simulink model "model"  (R2014a)
(part 8 of 8)

  _CN_242253500_500000_CN_204258596_500000/RConn3 -- T_204258596_500000_/LConn3 -- 関門連系線_CN_204258596_500000_CN_187988970_500000/RConn3 -- _CN_204258596_500000_CN_317416612_500000/RConn3 -- bus260/LConn1
  T_216956620_500000_/LConn1 -- 小丸川幹線_CN_216956620_500000_CN_216953915_220000/RConn1
  T_216956620_500000_/LConn2 -- 小丸川幹線_CN_216956620_500000_CN_216953915_220000/RConn2
  小丸川幹線_CN_216956620_500000_CN_216953915_220000/RConn3 -- T_216956620_500000_/LConn3 -- bus261/LConn1
  _CN_253566674_500000_CN_156208858_500000/LConn1 -- T_253566674__/LConn1 -- _CN_253566674_500000_CN_104391636_500000/LConn1
  _CN_253566674_500000_CN_156208858_500000/LConn2 -- T_253566674__/LConn2 -- _CN_253566674_500000_CN_104391636_500000/LConn2
  _CN_253566674_500000_CN_156208858_500000/LConn3 -- T_253566674__/LConn3 -- _CN_253566674_500000_CN_104391636_500000/LConn3 -- bus262/LConn1
  T_156208858_500000_南相馬変電所/LConn1 -- _CN_253566674_500000_CN_156208858_500000/RConn1
  T_156208858_500000_南相馬変電所/LConn2 -- _CN_253566674_500000_CN_156208858_500000/RConn2
  _CN_253566674_500000_CN_156208858_500000/RConn3 -- T_156208858_500000_南相馬変電所/LConn3 -- bus263/LConn1
  _CN_253566674_500000_CN_104391636_500000/RConn1 -- T_104391636_500000_新いわき/LConn1 -- 福島東幹線2_CN_106309481_500000_CN_104391636_500000/RConn1 -- _CN_132913106_500000_CN_104391636_500000/RConn1 -- 福島幹線_CN_104391636_500000_CN_168839127_500000/RConn1
  _CN_253566674_500000_CN_104391636_500000/RConn2 -- T_104391636_500000_新いわき/LConn2 -- 福島東幹線2_CN_106309481_500000_CN_104391636_500000/RConn2 -- _CN_132913106_500000_CN_104391636_500000/RConn2 -- 福島幹線_CN_104391636_500000_CN_168839127_500000/RConn2
  _CN_253566674_500000_CN_104391636_500000/RConn3 -- T_104391636_500000_新いわき/LConn3 -- 福島東幹線2_CN_106309481_500000_CN_104391636_500000/RConn3 -- _CN_132913106_500000_CN_104391636_500000/RConn3 -- 福島幹線_CN_104391636_500000_CN_168839127_500000/RConn3 -- bus264/LConn1
  新榛名線_CN_169963227_500000_CN_195615141_500000/LConn1 -- T_169963227_500000_新榛名/LConn1 -- _CN_169963227_500000_CN_169963236_500000/LConn1
  新榛名線_CN_169963227_500000_CN_195615141_500000/LConn2 -- T_169963227_500000_新榛名/LConn2 -- _CN_169963227_500000_CN_169963236_500000/LConn2
  新榛名線_CN_169963227_500000_CN_195615141_500000/LConn3 -- T_169963227_500000_新榛名/LConn3 -- _CN_169963227_500000_CN_169963236_500000/LConn3 -- bus265/LConn1
  新榛名線_CN_169963227_500000_CN_195615141_500000/RConn1 -- T_195615141_500000_/LConn1 -- _CN_195615141_500000_CN_315662839_500000/LConn1
  新榛名線_CN_169963227_500000_CN_195615141_500000/RConn2 -- T_195615141_500000_/LConn2 -- _CN_195615141_500000_CN_315662839_500000/LConn2
  新榛名線_CN_169963227_500000_CN_195615141_500000/RConn3 -- T_195615141_500000_/LConn3 -- _CN_195615141_500000_CN_315662839_500000/LConn3 -- bus266/LConn1
  _CN_169963227_500000_CN_169963236_500000/RConn1 -- T_169963236__/LConn1 -- 新吾妻線_CN_169963236_500000_CN_66098469_500000/RConn1
  _CN_169963227_500000_CN_169963236_500000/RConn2 -- T_169963236__/LConn2 -- 新吾妻線_CN_169963236_500000_CN_66098469_500000/RConn2
  _CN_169963227_500000_CN_169963236_500000/RConn3 -- T_169963236__/LConn3 -- 新吾妻線_CN_169963236_500000_CN_66098469_500000/RConn3 -- bus267/LConn1
  T_242103532_500000_/LConn1 -- _CN_242103532_500000_CN_241822623_500000/LConn1
  T_242103532_500000_/LConn2 -- _CN_242103532_500000_CN_241822623_500000/LConn2
  _CN_242103532_500000_CN_241822623_500000/LConn3 -- T_242103532_500000_/LConn3 -- bus268/LConn1
  _CN_242103532_500000_CN_241822623_500000/RConn1 -- T_241822623_500000;220000;110000_/LConn1 -- _CN_241822623_500000_CN_241822631_500000/LConn1 -- _CN_241828221_500000_CN_241822623_500000/RConn1
  _CN_242103532_500000_CN_241822623_500000/RConn2 -- T_241822623_500000;220000;110000_/LConn2 -- _CN_241822623_500000_CN_241822631_500000/LConn2 -- _CN_241828221_500000_CN_241822623_500000/RConn2
  _CN_242103532_500000_CN_241822623_500000/RConn3 -- T_241822623_500000;220000;110000_/LConn3 -- _CN_241822623_500000_CN_241822631_500000/LConn3 -- bus269/LConn1 -- _CN_241828221_500000_CN_241822623_500000/RConn3
  T_169031922__/LConn1 -- _CN_169031922_500000_CN_169031998_500000/LConn1
  T_169031922__/LConn2 -- _CN_169031922_500000_CN_169031998_500000/LConn2
  _CN_169031922_500000_CN_169031998_500000/LConn3 -- T_169031922__/LConn3 -- bus270/LConn1
  _CN_169031922_500000_CN_169031998_500000/RConn1 -- T_169031998__/LConn1 -- _CN_169031998_500000_CN_109850439_500000/LConn1 -- _CN_169031998_500000_CN_161870227_500000/RConn1
  _CN_169031922_500000_CN_169031998_500000/RConn2 -- T_169031998__/LConn2 -- _CN_169031998_500000_CN_109850439_500000/LConn2 -- _CN_169031998_500000_CN_161870227_500000/RConn2
  _CN_169031922_500000_CN_169031998_500000/RConn3 -- T_169031998__/LConn3 -- _CN_169031998_500000_CN_109850439_500000/LConn3 -- _CN_169031998_500000_CN_161870227_500000/RConn3 -- bus271/LConn1
  T_250540807_500000_東群馬変電所_(Higashi_Gunma_Substation)/LConn1 -- 東群馬幹線_CN_250540807_500000_CN_66098469_500000/RConn1
  T_250540807_500000_東群馬変電所_(Higashi_Gunma_Substation)/LConn2 -- 東群馬幹線_CN_250540807_500000_CN_66098469_500000/RConn2
  東群馬幹線_CN_250540807_500000_CN_66098469_500000/RConn3 -- T_250540807_500000_東群馬変電所_(Higashi_Gunma_Substation)/LConn3 -- bus272/LConn1
  T_151379730_500000_房総変電所_(Bōsō_Hendensho)/LConn1 -- 房総線_CN_151379730_500000_CN_168727982_500000/RConn1
  T_151379730_500000_房総変電所_(Bōsō_Hendensho)/LConn2 -- 房総線_CN_151379730_500000_CN_168727982_500000/RConn2
  房総線_CN_151379730_500000_CN_168727982_500000/RConn3 -- T_151379730_500000_房総変電所_(Bōsō_Hendensho)/LConn3 -- bus273/LConn1
  南信幹線_CN_142662111_500000_CN_209429410_500000/RConn1 -- T_209429410_500000_南信変電所/LConn1 -- 信濃幹線_CN_209726348_500000_CN_209429410_500000/LConn1
  南信幹線_CN_142662111_500000_CN_209429410_500000/RConn2 -- T_209429410_500000_南信変電所/LConn2 -- 信濃幹線_CN_209726348_500000_CN_209429410_500000/LConn2
  南信幹線_CN_142662111_500000_CN_209429410_500000/RConn3 -- T_209429410_500000_南信変電所/LConn3 -- 信濃幹線_CN_209726348_500000_CN_209429410_500000/LConn3 -- bus274/LConn1
  T_106076988_500000_宮城変電所/LConn1 -- _CN_106076988_500000_CN_174636874_500000/LConn1
  T_106076988_500000_宮城変電所/LConn2 -- _CN_106076988_500000_CN_174636874_500000/LConn2
  _CN_106076988_500000_CN_174636874_500000/LConn3 -- T_106076988_500000_宮城変電所/LConn3 -- bus275/LConn1
  T_174636874_275000_岩手変電所/LConn1 -- _CN_106076988_500000_CN_174636874_500000/RConn1
  T_174636874_275000_岩手変電所/LConn2 -- _CN_106076988_500000_CN_174636874_500000/RConn2
  _CN_106076988_500000_CN_174636874_500000/RConn3 -- T_174636874_275000_岩手変電所/LConn3 -- bus276/LConn1
  _CN_169031998_500000_CN_109850439_500000/RConn1 -- T_109850439_500000_/LConn1 -- 阿南紀北直流幹線_CN_109850439_500000_CN_217885658_500000/LConn1
  _CN_169031998_500000_CN_109850439_500000/RConn2 -- T_109850439_500000_/LConn2 -- 阿南紀北直流幹線_CN_109850439_500000_CN_217885658_500000/LConn2
  _CN_169031998_500000_CN_109850439_500000/RConn3 -- T_109850439_500000_/LConn3 -- 阿南紀北直流幹線_CN_109850439_500000_CN_217885658_500000/LConn3 -- bus277/LConn1
  新筑波線_(Shin_Tsukuba_Sen)_CN_133135172_500000_CN_132913106_500000/RConn1 -- T_133135172_500000_新古河変電所/LConn1 -- 新京葉線_CN_133135172_500000_CN_168727982_500000/RConn1 -- 新京葉線_CN_133135172_500000_CN_151706977_500000/LConn1 -- 新古河線_(Shin_Koga_Sen)_CN_133135172_500000_CN_133641619_500000/RConn1 -- 福島幹線_CN_133135172_500000_CN_168839127_500000/RConn1
  新筑波線_(Shin_Tsukuba_Sen)_CN_133135172_500000_CN_132913106_500000/RConn2 -- T_133135172_500000_新古河変電所/LConn2 -- 新京葉線_CN_133135172_500000_CN_168727982_500000/RConn2 -- 新京葉線_CN_133135172_500000_CN_151706977_500000/LConn2 -- 新古河線_(Shin_Koga_Sen)_CN_133135172_500000_CN_133641619_500000/RConn2 -- 福島幹線_CN_133135172_500000_CN_168839127_500000/RConn2
  新筑波線_(Shin_Tsukuba_Sen)_CN_133135172_500000_CN_132913106_500000/RConn3 -- T_133135172_500000_新古河変電所/LConn3 -- 新京葉線_CN_133135172_500000_CN_168727982_500000/RConn3 -- 新京葉線_CN_133135172_500000_CN_151706977_500000/LConn3 -- 新古河線_(Shin_Koga_Sen)_CN_133135172_500000_CN_133641619_500000/RConn3 -- 福島幹線_CN_133135172_500000_CN_168839127_500000/RConn3 -- bus278/LConn1
  T_151706977__新野田変電所_(Shin_Noda_Hendensho)/LConn1 -- 新京葉線_CN_133135172_500000_CN_151706977_500000/RConn1
  T_151706977__新野田変電所_(Shin_Noda_Hendensho)/LConn2 -- 新京葉線_CN_133135172_500000_CN_151706977_500000/RConn2
  新京葉線_CN_133135172_500000_CN_151706977_500000/RConn3 -- T_151706977__新野田変電所_(Shin_Noda_Hendensho)/LConn3 -- bus279/LConn1
  T_217885658_500000;0_由良開閉所/LConn1 -- 阿南紀北直流幹線_CN_109850439_500000_CN_217885658_500000/RConn1
  T_217885658_500000;0_由良開閉所/LConn2 -- 阿南紀北直流幹線_CN_109850439_500000_CN_217885658_500000/RConn2
  阿南紀北直流幹線_CN_109850439_500000_CN_217885658_500000/RConn3 -- T_217885658_500000;0_由良開閉所/LConn3 -- bus280/LConn1
  T_185029969_500000;220000_/LConn1 -- _CN_185029969_500000_CN_216798219_500000/LConn1
  T_185029969_500000;220000_/LConn2 -- _CN_185029969_500000_CN_216798219_500000/LConn2
  _CN_185029969_500000_CN_216798219_500000/LConn3 -- T_185029969_500000;220000_/LConn3 -- bus281/LConn1
  G_216798219_九州電力_松浦火力発電所/RConn1 -- _CN_185029969_500000_CN_216798219_500000/RConn1
  G_216798219_九州電力_松浦火力発電所/RConn2 -- _CN_185029969_500000_CN_216798219_500000/RConn2
  _CN_185029969_500000_CN_216798219_500000/RConn3 -- G_216798219_九州電力_松浦火力発電所/RConn3 -- bus282/LConn1
  _CN_170605907_500000_CN_110682956_500000/RConn1 -- T_170605907_500000_北摂変電所/LConn1 -- _CN_170605907_500000_CN_241822631_500000/LConn1
  _CN_170605907_500000_CN_110682956_500000/RConn2 -- T_170605907_500000_北摂変電所/LConn2 -- _CN_170605907_500000_CN_241822631_500000/LConn2
  _CN_170605907_500000_CN_110682956_500000/RConn3 -- T_170605907_500000_北摂変電所/LConn3 -- _CN_170605907_500000_CN_241822631_500000/LConn3 -- bus283/LConn1
  _CN_170605907_500000_CN_241822631_500000/RConn1 -- T_241822631__/LConn1 -- _CN_241822623_500000_CN_241822631_500000/RConn1 -- _CN_241822621_500000_CN_241822631_500000/RConn1
  _CN_170605907_500000_CN_241822631_500000/RConn2 -- T_241822631__/LConn2 -- _CN_241822623_500000_CN_241822631_500000/RConn2 -- _CN_241822621_500000_CN_241822631_500000/RConn2
  _CN_170605907_500000_CN_241822631_500000/RConn3 -- T_241822631__/LConn3 -- _CN_241822623_500000_CN_241822631_500000/RConn3 -- bus284/LConn1 -- _CN_241822621_500000_CN_241822631_500000/RConn3
  T_209726348_500000_信濃変電所/LConn1 -- 信濃幹線_CN_209726348_500000_CN_209429410_500000/RConn1
  T_209726348_500000_信濃変電所/LConn2 -- 信濃幹線_CN_209726348_500000_CN_209429410_500000/RConn2
  信濃幹線_CN_209726348_500000_CN_209429410_500000/RConn3 -- T_209726348_500000_信濃変電所/LConn3 -- bus285/LConn1
  T_315662839_500000_新信濃変電所/LConn1 -- _CN_195615141_500000_CN_315662839_500000/RConn1
  T_315662839_500000_新信濃変電所/LConn2 -- _CN_195615141_500000_CN_315662839_500000/RConn2
  _CN_195615141_500000_CN_315662839_500000/RConn3 -- T_315662839_500000_新信濃変電所/LConn3 -- bus286/LConn1
  T_259056356__/RConn1 -- L_259056356/LConn1
  T_259056356__/RConn2 -- L_259056356/LConn2
  L_259056356/LConn3 -- T_259056356__/RConn3 -- bus287/LConn1
  T_90806466_220000;66000_/RConn1 -- L_90806466/LConn1
  T_90806466_220000;66000_/RConn2 -- L_90806466/LConn2
  L_90806466/LConn3 -- T_90806466_220000;66000_/RConn3 -- bus288/LConn1
  T_216498433_220000;110000;66000_九州電力_南熊本変電所/RConn1 -- L_216498433/LConn1
  T_216498433_220000;110000;66000_九州電力_南熊本変電所/RConn2 -- L_216498433/LConn2
  L_216498433/LConn3 -- T_216498433_220000;110000;66000_九州電力_南熊本変電所/RConn3 -- bus289/LConn1
  T_203776442__/RConn1 -- L_203776442/LConn1
  T_203776442__/RConn2 -- L_203776442/LConn2
  L_203776442/LConn3 -- T_203776442__/RConn3 -- bus290/LConn1
  T_216496817_220000;66000_九州電力人吉変電所/RConn1 -- L_216496817/LConn1
  T_216496817_220000;66000_九州電力人吉変電所/RConn2 -- L_216496817/LConn2
  L_216496817/LConn3 -- T_216496817_220000;66000_九州電力人吉変電所/RConn3 -- bus291/LConn1
  T_373882198__/RConn1 -- L_373882198/LConn1
  T_373882198__/RConn2 -- L_373882198/LConn2
  L_373882198/LConn3 -- T_373882198__/RConn3 -- bus292/LConn1
  T_218035208_220000_高野変電所/RConn1 -- L_218035208/LConn1
  T_218035208_220000_高野変電所/RConn2 -- L_218035208/LConn2
  L_218035208/LConn3 -- T_218035208_220000_高野変電所/RConn3 -- bus293/LConn1
  T_189776902_220000;66000_九州電力_門司変電所/RConn1 -- L_189776902/LConn1
  T_189776902_220000;66000_九州電力_門司変電所/RConn2 -- L_189776902/LConn2
  L_189776902/LConn3 -- T_189776902_220000;66000_九州電力_門司変電所/RConn3 -- bus294/LConn1
  T_296958054_220000;25000_JR西日本_新門司変電所/RConn1 -- L_296958054/LConn1
  T_296958054_220000;25000_JR西日本_新門司変電所/RConn2 -- L_296958054/LConn2
  L_296958054/LConn3 -- T_296958054_220000;25000_JR西日本_新門司変電所/RConn3 -- bus295/LConn1
  T_405705606_220000;66000_/RConn1 -- L_405705606/LConn1
  T_405705606_220000;66000_/RConn2 -- L_405705606/LConn2
  L_405705606/LConn3 -- T_405705606_220000;66000_/RConn3 -- bus296/LConn1
  T_239024744_220000;110000;66000_九州電力_西谷変電所/RConn1 -- L_239024744/LConn1
  T_239024744_220000;110000;66000_九州電力_西谷変電所/RConn2 -- L_239024744/LConn2
  L_239024744/LConn3 -- T_239024744_220000;110000;66000_九州電力_西谷変電所/RConn3 -- bus297/LConn1
  T_317951887_500000_/RConn1 -- L_317951887/LConn1
  T_317951887_500000_/RConn2 -- L_317951887/LConn2
  L_317951887/LConn3 -- T_317951887_500000_/RConn3 -- bus298/LConn1
  T_170974372_220000;110000_広島変電所/RConn1 -- L_170974372/LConn1
  T_170974372_220000;110000_広島変電所/RConn2 -- L_170974372/LConn2
  L_170974372/LConn3 -- T_170974372_220000;110000_広島変電所/RConn3 -- bus299/LConn1
  T_317980483_220000_/RConn1 -- L_317980483/LConn1
  T_317980483_220000_/RConn2 -- L_317980483/LConn2
  L_317980483/LConn3 -- T_317980483_220000_/RConn3 -- bus300/LConn1
  T_319463514_220000;110000_下松発電所/RConn1 -- L_319463514/LConn1
  T_319463514_220000;110000_下松発電所/RConn2 -- L_319463514/LConn2
  L_319463514/LConn3 -- T_319463514_220000;110000_下松発電所/RConn3 -- bus301/LConn1
  T_243471278_220000_/RConn1 -- L_243471278/LConn1
  T_243471278_220000_/RConn2 -- L_243471278/LConn2
  L_243471278/LConn3 -- T_243471278_220000_/RConn3 -- bus302/LConn1
  T_406052986_220000_/RConn1 -- L_406052986/LConn1
  T_406052986_220000_/RConn2 -- L_406052986/LConn2
  L_406052986/LConn3 -- T_406052986_220000_/RConn3 -- bus303/LConn1
  T_242159178_220000_/RConn1 -- L_242159178/LConn1
  T_242159178_220000_/RConn2 -- L_242159178/LConn2
  L_242159178/LConn3 -- T_242159178_220000_/RConn3 -- bus304/LConn1
  T_373870139__/RConn1 -- L_373870139/LConn1
  T_373870139__/RConn2 -- L_373870139/LConn2
  L_373870139/LConn3 -- T_373870139__/RConn3 -- bus305/LConn1
  T_173152424_220000;66000_九州電力_西福岡変電所/RConn1 -- L_173152424/LConn1
  T_173152424_220000;66000_九州電力_西福岡変電所/RConn2 -- L_173152424/LConn2
  L_173152424/LConn3 -- T_173152424_220000;66000_九州電力_西福岡変電所/RConn3 -- bus306/LConn1
  T_238089516_220000_九州新幹線_新鳥栖変電所/RConn1 -- L_238089516/LConn1
  T_238089516_220000_九州新幹線_新鳥栖変電所/RConn2 -- L_238089516/LConn2
  L_238089516/LConn3 -- T_238089516_220000_九州新幹線_新鳥栖変電所/RConn3 -- bus307/LConn1
  T_173793392__鳥栖変電所/RConn1 -- L_173793392/LConn1
  T_173793392__鳥栖変電所/RConn2 -- L_173793392/LConn2
  L_173793392/LConn3 -- T_173793392__鳥栖変電所/RConn3 -- bus308/LConn1
  T_319371122_220000_/RConn1 -- L_319371122/LConn1
  T_319371122_220000_/RConn2 -- L_319371122/LConn2
  L_319371122/LConn3 -- T_319371122_220000_/RConn3 -- bus309/LConn1
  T_318438125_220000_/RConn1 -- L_318438125/LConn1
  T_318438125_220000_/RConn2 -- L_318438125/LConn2
  L_318438125/LConn3 -- T_318438125_220000_/RConn3 -- bus310/LConn1
  T_172143432__/RConn1 -- L_172143432/LConn1
  T_172143432__/RConn2 -- L_172143432/LConn2
  L_172143432/LConn3 -- T_172143432__/RConn3 -- bus311/LConn1
  T_184180157_220000;66000_東福岡変電所/RConn1 -- L_184180157/LConn1
  T_184180157_220000;66000_東福岡変電所/RConn2 -- L_184180157/LConn2
  L_184180157/LConn3 -- T_184180157_220000;66000_東福岡変電所/RConn3 -- bus312/LConn1
  T_405806514_220000;66000_/RConn1 -- L_405806514/LConn1
  T_405806514_220000;66000_/RConn2 -- L_405806514/LConn2
  L_405806514/LConn3 -- T_405806514_220000;66000_/RConn3 -- bus313/LConn1
  T_189777972__/RConn1 -- L_189777972/LConn1
  T_189777972__/RConn2 -- L_189777972/LConn2
  L_189777972/LConn3 -- T_189777972__/RConn3 -- bus314/LConn1
  T_296789326__/RConn1 -- L_296789326/LConn1
  T_296789326__/RConn2 -- L_296789326/LConn2
  L_296789326/LConn3 -- T_296789326__/RConn3 -- bus315/LConn1
  T_201289289_220000_九州電力_唐津変電所/RConn1 -- L_201289289/LConn1
  T_201289289_220000_九州電力_唐津変電所/RConn2 -- L_201289289/LConn2
  L_201289289/LConn3 -- T_201289289_220000_九州電力_唐津変電所/RConn3 -- bus316/LConn1
  T_174915836_220000;66000_九州電力_木佐木変電所/RConn1 -- L_174915836/LConn1
  T_174915836_220000;66000_九州電力_木佐木変電所/RConn2 -- L_174915836/LConn2
  L_174915836/LConn3 -- T_174915836_220000;66000_九州電力_木佐木変電所/RConn3 -- bus317/LConn1
  T_216949339_220000;110000;66000_/RConn1 -- L_216949339/LConn1
  T_216949339_220000;110000;66000_/RConn2 -- L_216949339/LConn2
  L_216949339/LConn3 -- T_216949339_220000;110000;66000_/RConn3 -- bus318/LConn1
  T_186510275_500000_3_4号_開閉所/RConn1 -- L_186510275/LConn1
  T_186510275_500000_3_4号_開閉所/RConn2 -- L_186510275/LConn2
  L_186510275/LConn3 -- T_186510275_500000_3_4号_開閉所/RConn3 -- bus319/LConn1
  T_220698807__/RConn1 -- L_220698807/LConn1
  T_220698807__/RConn2 -- L_220698807/LConn2
  L_220698807/LConn3 -- T_220698807__/RConn3 -- bus320/LConn1
  T_219579624_220000_/RConn1 -- L_219579624/LConn1
  T_219579624_220000_/RConn2 -- L_219579624/LConn2
  L_219579624/LConn3 -- T_219579624_220000_/RConn3 -- bus321/LConn1
  T_241875111_220000_/RConn1 -- L_241875111/LConn1
  T_241875111_220000_/RConn2 -- L_241875111/LConn2
  L_241875111/LConn3 -- T_241875111_220000_/RConn3 -- bus322/LConn1
  T_185504478_220000;66000_/RConn1 -- L_185504478/LConn1
  T_185504478_220000;66000_/RConn2 -- L_185504478/LConn2
  L_185504478/LConn3 -- T_185504478_220000;66000_/RConn3 -- bus323/LConn1
  T_242389846__/RConn1 -- L_242389846/LConn1
  T_242389846__/RConn2 -- L_242389846/LConn2
  L_242389846/LConn3 -- T_242389846__/RConn3 -- bus324/LConn1
  T_172144358_500000;220000_/RConn1 -- L_172144358/LConn1
  T_172144358_500000;220000_/RConn2 -- L_172144358/LConn2
  L_172144358/LConn3 -- T_172144358_500000;220000_/RConn3 -- bus325/LConn1
  T_172144359_500000;220000_/RConn1 -- L_172144359/LConn1
  T_172144359_500000;220000_/RConn2 -- L_172144359/LConn2
  L_172144359/LConn3 -- T_172144359_500000;220000_/RConn3 -- bus326/LConn1
  T_297939963_220000_/RConn1 -- L_297939963/LConn1
  T_297939963_220000_/RConn2 -- L_297939963/LConn2
  L_297939963/LConn3 -- T_297939963_220000_/RConn3 -- bus327/LConn1
  T_296788490_220000;66000_九州電力_上津役変電所/RConn1 -- L_296788490/LConn1
  T_296788490_220000;66000_九州電力_上津役変電所/RConn2 -- L_296788490/LConn2
  L_296788490/LConn3 -- T_296788490_220000;66000_九州電力_上津役変電所/RConn3 -- bus328/LConn1
  T_238813045_220000_/RConn1 -- L_238813045/LConn1
  T_238813045_220000_/RConn2 -- L_238813045/LConn2
  L_238813045/LConn3 -- T_238813045_220000_/RConn3 -- bus329/LConn1
  T_238813048_220000_出水変電所/RConn1 -- L_238813048/LConn1
  T_238813048_220000_出水変電所/RConn2 -- L_238813048/LConn2
  L_238813048/LConn3 -- T_238813048_220000_出水変電所/RConn3 -- bus330/LConn1
  T_237475191_220000_九州電力_新鹿児島変電所/RConn1 -- L_237475191/LConn1
  T_237475191_220000_九州電力_新鹿児島変電所/RConn2 -- L_237475191/LConn2
  L_237475191/LConn3 -- T_237475191_220000_九州電力_新鹿児島変電所/RConn3 -- bus331/LConn1
  T_169121281__北豊田変電所_(Kita_Toyota_Hendensho)/RConn1 -- L_169121281/LConn1
  T_169121281__北豊田変電所_(Kita_Toyota_Hendensho)/RConn2 -- L_169121281/LConn2
  L_169121281/LConn3 -- T_169121281__北豊田変電所_(Kita_Toyota_Hendensho)/RConn3 -- bus332/LConn1
  T_169121284_275000_/RConn1 -- L_169121284/LConn1
  T_169121284_275000_/RConn2 -- L_169121284/LConn2
  L_169121284/LConn3 -- T_169121284_275000_/RConn3 -- bus333/LConn1
  T_116828675_275000_北相模変電所_(Kita_Sagami_Hendensho)/RConn1 -- L_116828675/LConn1
  T_116828675_275000_北相模変電所_(Kita_Sagami_Hendensho)/RConn2 -- L_116828675/LConn2
  L_116828675/LConn3 -- T_116828675_275000_北相模変電所_(Kita_Sagami_Hendensho)/RConn3 -- bus334/LConn1
  T_169121278_275000_電源名古屋/RConn1 -- L_169121278/LConn1
  T_169121278_275000_電源名古屋/RConn2 -- L_169121278/LConn2
  L_169121278/LConn3 -- T_169121278_275000_電源名古屋/RConn3 -- bus335/LConn1
  T_170503689__駿遠変電所/RConn1 -- L_170503689/LConn1
  T_170503689__駿遠変電所/RConn2 -- L_170503689/LConn2
  L_170503689/LConn3 -- T_170503689__駿遠変電所/RConn3 -- bus336/LConn1
  T_170436908__/RConn1 -- L_170436908/LConn1
  T_170436908__/RConn2 -- L_170436908/LConn2
  L_170436908/LConn3 -- T_170436908__/RConn3 -- bus337/LConn1
  T_158064651_275000_田子倉発電所/RConn1 -- L_158064651/LConn1
  T_158064651_275000_田子倉発電所/RConn2 -- L_158064651/LConn2
  L_158064651/LConn3 -- T_158064651_275000_田子倉発電所/RConn3 -- bus338/LConn1
  T_232998815_275000_/RConn1 -- L_232998815/LConn1
  T_232998815_275000_/RConn2 -- L_232998815/LConn2
  L_232998815/LConn3 -- T_232998815_275000_/RConn3 -- bus339/LConn1
  T_241956440_275000_伊勢開閉所/RConn1 -- L_241956440/LConn1
  T_241956440_275000_伊勢開閉所/RConn2 -- L_241956440/LConn2
  L_241956440/LConn3 -- T_241956440_275000_伊勢開閉所/RConn3 -- bus340/LConn1
  T_241923317_275000_南勢変電所_(Nansei_Hendensho)/RConn1 -- L_241923317/LConn1
  T_241923317_275000_南勢変電所_(Nansei_Hendensho)/RConn2 -- L_241923317/LConn2
  L_241923317/LConn3 -- T_241923317_275000_南勢変電所_(Nansei_Hendensho)/RConn3 -- bus341/LConn1
  T_242532736_275000_/RConn1 -- L_242532736/LConn1
  T_242532736_275000_/RConn2 -- L_242532736/LConn2
  L_242532736/LConn3 -- T_242532736_275000_/RConn3 -- bus342/LConn1
  T_162844704_275000_中相模変電所/RConn1 -- L_162844704/LConn1
  T_162844704_275000_中相模変電所/RConn2 -- L_162844704/LConn2
  L_162844704/LConn3 -- T_162844704_275000_中相模変電所/RConn3 -- bus343/LConn1
  T_128364781_275000_東京電力_京浜変電所/RConn1 -- L_128364781/LConn1
  T_128364781_275000_東京電力_京浜変電所/RConn2 -- L_128364781/LConn2
  L_128364781/LConn3 -- T_128364781_275000_東京電力_京浜変電所/RConn3 -- bus344/LConn1
  T_210765350__花見川変電所_(Hanamigawa_Hendensho)/RConn1 -- L_210765350/LConn1
  T_210765350__花見川変電所_(Hanamigawa_Hendensho)/RConn2 -- L_210765350/LConn2
  L_210765350/LConn3 -- T_210765350__花見川変電所_(Hanamigawa_Hendensho)/RConn3 -- bus345/LConn1
  T_211241774__/RConn1 -- L_211241774/LConn1
  T_211241774__/RConn2 -- L_211241774/LConn2
  L_211241774/LConn3 -- T_211241774__/RConn3 -- bus346/LConn1
  T_179863079_275000_/RConn1 -- L_179863079/LConn1
  T_179863079_275000_/RConn2 -- L_179863079/LConn2
  L_179863079/LConn3 -- T_179863079_275000_/RConn3 -- bus347/LConn1
  T_256894928__/RConn1 -- L_256894928/LConn1
  T_256894928__/RConn2 -- L_256894928/LConn2
  L_256894928/LConn3 -- T_256894928__/RConn3 -- bus348/LConn1
  T_168524732__/RConn1 -- L_168524732/LConn1
  T_168524732__/RConn2 -- L_168524732/LConn2
  L_168524732/LConn3 -- T_168524732__/RConn3 -- bus349/LConn1
  T_319300956_275000_中越変電所/RConn1 -- L_319300956/LConn1
  T_319300956_275000_中越変電所/RConn2 -- L_319300956/LConn2
  L_319300956/LConn3 -- T_319300956_275000_中越変電所/RConn3 -- bus350/LConn1
  T_318218831_275000_/RConn1 -- L_318218831/LConn1
  T_318218831_275000_/RConn2 -- L_318218831/LConn2
  L_318218831/LConn3 -- T_318218831_275000_/RConn3 -- bus351/LConn1
  T_161948515_275000_西濃変電所_(Seinō_Hendensho)/RConn1 -- L_161948515/LConn1
  T_161948515_275000_西濃変電所_(Seinō_Hendensho)/RConn2 -- L_161948515/LConn2
  L_161948515/LConn3 -- T_161948515_275000_西濃変電所_(Seinō_Hendensho)/RConn3 -- bus352/LConn1
  T_170793702_275000_西名古屋/RConn1 -- L_170793702/LConn1
  T_170793702_275000_西名古屋/RConn2 -- L_170793702/LConn2
  L_170793702/LConn3 -- T_170793702_275000_西名古屋/RConn3 -- bus353/LConn1
  T_170793703_275000_西尾張/RConn1 -- L_170793703/LConn1
  T_170793703_275000_西尾張/RConn2 -- L_170793703/LConn2
  L_170793703/LConn3 -- T_170793703_275000_西尾張/RConn3 -- bus354/LConn1
  T_340647468__/RConn1 -- L_340647468/LConn1
  T_340647468__/RConn2 -- L_340647468/LConn2
  L_340647468/LConn3 -- T_340647468__/RConn3 -- bus355/LConn1
  T_340648895__/RConn1 -- L_340648895/LConn1
  T_340648895__/RConn2 -- L_340648895/LConn2
  L_340648895/LConn3 -- T_340648895__/RConn3 -- bus356/LConn1
  T_168852840__/RConn1 -- L_168852840/LConn1
  T_168852840__/RConn2 -- L_168852840/LConn2
  L_168852840/LConn3 -- T_168852840__/RConn3 -- bus357/LConn1
  T_192745005_275000_丸山変電所_(Maruyama_Hendensho)/RConn1 -- L_192745005/LConn1
  T_192745005_275000_丸山変電所_(Maruyama_Hendensho)/RConn2 -- L_192745005/LConn2
  L_192745005/LConn3 -- T_192745005_275000_丸山変電所_(Maruyama_Hendensho)/RConn3 -- bus358/LConn1
  T_161946848_275000_関開閉所_(Seki)/RConn1 -- L_161946848/LConn1
  T_161946848_275000_関開閉所_(Seki)/RConn2 -- L_161946848/LConn2
  L_161946848/LConn3 -- T_161946848_275000_関開閉所_(Seki)/RConn3 -- bus359/LConn1
  T_168903220_275000_/RConn1 -- L_168903220/LConn1
  T_168903220_275000_/RConn2 -- L_168903220/LConn2
  L_168903220/LConn3 -- T_168903220_275000_/RConn3 -- bus360/LConn1
  T_315434352__/RConn1 -- L_315434352/LConn1
  T_315434352__/RConn2 -- L_315434352/LConn2
  L_315434352/LConn3 -- T_315434352__/RConn3 -- bus361/LConn1
  T_315434358_500000_新岡部変電所/RConn1 -- L_315434358/LConn1
  T_315434358_500000_新岡部変電所/RConn2 -- L_315434358/LConn2
  L_315434358/LConn3 -- T_315434358_500000_新岡部変電所/RConn3 -- bus362/LConn1
  T_108199478_275000_南大阪変電所_(Minamiōsaka_Hendensho)/RConn1 -- L_108199478/LConn1
  T_108199478_275000_南大阪変電所_(Minamiōsaka_Hendensho)/RConn2 -- L_108199478/LConn2
  L_108199478/LConn3 -- T_108199478_275000_南大阪変電所_(Minamiōsaka_Hendensho)/RConn3 -- bus363/LConn1
  T_158522649_275000_東大阪変電所/RConn1 -- L_158522649/LConn1
  T_158522649_275000_東大阪変電所/RConn2 -- L_158522649/LConn2
  L_158522649/LConn3 -- T_158522649_275000_東大阪変電所/RConn3 -- bus364/LConn1
  T_109834508_275000_金剛開閉所_(Kongō_Kaiheisho)/RConn1 -- L_109834508/LConn1
  T_109834508_275000_金剛開閉所_(Kongō_Kaiheisho)/RConn2 -- L_109834508/LConn2
  L_109834508/LConn3 -- T_109834508_275000_金剛開閉所_(Kongō_Kaiheisho)/RConn3 -- bus365/LConn1
  T_315614776_275000_/RConn1 -- L_315614776/LConn1
  T_315614776_275000_/RConn2 -- L_315614776/LConn2
  L_315614776/LConn3 -- T_315614776_275000_/RConn3 -- bus366/LConn1
  T_315614783_275000_/RConn1 -- L_315614783/LConn1
  T_315614783_275000_/RConn2 -- L_315614783/LConn2
  L_315614783/LConn3 -- T_315614783_275000_/RConn3 -- bus367/LConn1
  T_316566585_275000_/RConn1 -- L_316566585/LConn1
  T_316566585_275000_/RConn2 -- L_316566585/LConn2
  L_316566585/LConn3 -- T_316566585_275000_/RConn3 -- bus368/LConn1
  T_316566588_275000_/RConn1 -- L_316566588/LConn1
  T_316566588_275000_/RConn2 -- L_316566588/LConn2
  L_316566588/LConn3 -- T_316566588_275000_/RConn3 -- bus369/LConn1
  T_316581632_275000_/RConn1 -- L_316581632/LConn1
  T_316581632_275000_/RConn2 -- L_316581632/LConn2
  L_316581632/LConn3 -- T_316581632_275000_/RConn3 -- bus370/LConn1
  T_256682313__/RConn1 -- L_256682313/LConn1
  T_256682313__/RConn2 -- L_256682313/LConn2
  L_256682313/LConn3 -- T_256682313__/RConn3 -- bus371/LConn1
  T_103818820_275000_仙台変電所/RConn1 -- L_103818820/LConn1
  T_103818820_275000_仙台変電所/RConn2 -- L_103818820/LConn2
  L_103818820/LConn3 -- T_103818820_275000_仙台変電所/RConn3 -- bus372/LConn1
  T_250430935_275000_米沢変電所_(Yonezawa_Hendensho)/RConn1 -- L_250430935/LConn1
  T_250430935_275000_米沢変電所_(Yonezawa_Hendensho)/RConn2 -- L_250430935/LConn2
  L_250430935/LConn3 -- T_250430935_275000_米沢変電所_(Yonezawa_Hendensho)/RConn3 -- bus373/LConn1
  T_170693194_275000_淀川/RConn1 -- L_170693194/LConn1
  T_170693194_275000_淀川/RConn2 -- L_170693194/LConn2
  L_170693194/LConn3 -- T_170693194_275000_淀川/RConn3 -- bus374/LConn1
  T_169993955_275000_新潟変電所/RConn1 -- L_169993955/LConn1
  T_169993955_275000_新潟変電所/RConn2 -- L_169993955/LConn2
  L_169993955/LConn3 -- T_169993955_275000_新潟変電所/RConn3 -- bus375/LConn1
  T_170016148_275000_北新潟変電所/RConn1 -- L_170016148/LConn1
  T_170016148_275000_北新潟変電所/RConn2 -- L_170016148/LConn2
  L_170016148/LConn3 -- T_170016148_275000_北新潟変電所/RConn3 -- bus376/LConn1
  T_170247359_275000_/RConn1 -- L_170247359/LConn1
  T_170247359_275000_/RConn2 -- L_170247359/LConn2
  L_170247359/LConn3 -- T_170247359_275000_/RConn3 -- bus377/LConn1
  T_179417733_275000_/RConn1 -- L_179417733/LConn1
  T_179417733_275000_/RConn2 -- L_179417733/LConn2
  L_179417733/LConn3 -- T_179417733_275000_/RConn3 -- bus378/LConn1
  T_170366038_275000_/RConn1 -- L_170366038/LConn1
  T_170366038_275000_/RConn2 -- L_170366038/LConn2
  L_170366038/LConn3 -- T_170366038_275000_/RConn3 -- bus379/LConn1
  T_170366039__中部電力遠江変電所/RConn1 -- L_170366039/LConn1
  T_170366039__中部電力遠江変電所/RConn2 -- L_170366039/LConn2
  L_170366039/LConn3 -- T_170366039__中部電力遠江変電所/RConn3 -- bus380/LConn1
  T_104375141_275000_須賀川変電所_(Sukagawa_Hendensho)/RConn1 -- L_104375141/LConn1
  T_104375141_275000_須賀川変電所_(Sukagawa_Hendensho)/RConn2 -- L_104375141/LConn2
  L_104375141/LConn3 -- T_104375141_275000_須賀川変電所_(Sukagawa_Hendensho)/RConn3 -- bus381/LConn1
  T_107262429_275000_福島変電所/RConn1 -- L_107262429/LConn1
  T_107262429_275000_福島変電所/RConn2 -- L_107262429/LConn2
  L_107262429/LConn3 -- T_107262429_275000_福島変電所/RConn3 -- bus382/LConn1
  T_262597734__海部開閉所/RConn1 -- L_262597734/LConn1
  T_262597734__海部開閉所/RConn2 -- L_262597734/LConn2
  L_262597734/LConn3 -- T_262597734__海部開閉所/RConn3 -- bus383/LConn1
  T_315757225_275000_/RConn1 -- L_315757225/LConn1
  T_315757225_275000_/RConn2 -- L_315757225/LConn2
  L_315757225/LConn3 -- T_315757225_275000_/RConn3 -- bus384/LConn1
  T_87682157_275000_南川越変電所_(Minamikawagoe_Hendensho)/RConn1 -- L_87682157/LConn1
  T_87682157_275000_南川越変電所_(Minamikawagoe_Hendensho)/RConn2 -- L_87682157/LConn2
  L_87682157/LConn3 -- T_87682157_275000_南川越変電所_(Minamikawagoe_Hendensho)/RConn3 -- bus385/LConn1
  T_159491797_275000_南狭山変電所_(Minamisayama_Hendensho)/RConn1 -- L_159491797/LConn1
  T_159491797_275000_南狭山変電所_(Minamisayama_Hendensho)/RConn2 -- L_159491797/LConn2
  L_159491797/LConn3 -- T_159491797_275000_南狭山変電所_(Minamisayama_Hendensho)/RConn3 -- bus386/LConn1
  T_105291887_275000_那珂変電所_(Naka_Hendensho)/RConn1 -- L_105291887/LConn1
  T_105291887_275000_那珂変電所_(Naka_Hendensho)/RConn2 -- L_105291887/LConn2
  L_105291887/LConn3 -- T_105291887_275000_那珂変電所_(Naka_Hendensho)/RConn3 -- bus387/LConn1
  T_155411568__/RConn1 -- L_155411568/LConn1
  T_155411568__/RConn2 -- L_155411568/LConn2
  L_155411568/LConn3 -- T_155411568__/RConn3 -- bus388/LConn1
  T_153521822_275000_西越谷変電所_(Nishi_Koshigaya_Hendensho)/RConn1 -- L_153521822/LConn1
  T_153521822_275000_西越谷変電所_(Nishi_Koshigaya_Hendensho)/RConn2 -- L_153521822/LConn2
  L_153521822/LConn3 -- T_153521822_275000_西越谷変電所_(Nishi_Koshigaya_Hendensho)/RConn3 -- bus389/LConn1
  T_133137636_275000_北東京変電所_(Kita_Tōkyō_Hendensho)/RConn1 -- L_133137636/LConn1
  T_133137636_275000_北東京変電所_(Kita_Tōkyō_Hendensho)/RConn2 -- L_133137636/LConn2
  L_133137636/LConn3 -- T_133137636_275000_北東京変電所_(Kita_Tōkyō_Hendensho)/RConn3 -- bus390/LConn1
  T_316796028_275000_/RConn1 -- L_316796028/LConn1
  T_316796028_275000_/RConn2 -- L_316796028/LConn2
  L_316796028/LConn3 -- T_316796028_275000_/RConn3 -- bus391/LConn1
  T_170247308_275000_三河変電所/RConn1 -- L_170247308/LConn1
  T_170247308_275000_三河変電所/RConn2 -- L_170247308/LConn2
  L_170247308/LConn3 -- T_170247308_275000_三河変電所/RConn3 -- bus392/LConn1
  T_170260165_275000_中部電力湖西変電所/RConn1 -- L_170260165/LConn1
  T_170260165_275000_中部電力湖西変電所/RConn2 -- L_170260165/LConn2
  L_170260165/LConn3 -- T_170260165_275000_中部電力湖西変電所/RConn3 -- bus393/LConn1
  T_170247314_275000_額田開閉所/RConn1 -- L_170247314/LConn1
  T_170247314_275000_額田開閉所/RConn2 -- L_170247314/LConn2
  L_170247314/LConn3 -- T_170247314_275000_額田開閉所/RConn3 -- bus394/LConn1
  T_302164677__秋田変電所/RConn1 -- L_302164677/LConn1
  T_302164677__秋田変電所/RConn2 -- L_302164677/LConn2
  L_302164677/LConn3 -- T_302164677__秋田変電所/RConn3 -- bus395/LConn1
  T_302164679_275000_能代変電所/RConn1 -- L_302164679/LConn1
  T_302164679_275000_能代変電所/RConn2 -- L_302164679/LConn2
  L_302164679/LConn3 -- T_302164679_275000_能代変電所/RConn3 -- bus396/LConn1
  T_316727625_275000_/RConn1 -- L_316727625/LConn1
  T_316727625_275000_/RConn2 -- L_316727625/LConn2
  L_316727625/LConn3 -- T_316727625_275000_/RConn3 -- bus397/LConn1
  T_316581637_275000_青森変電所/RConn1 -- L_316581637/LConn1
  T_316581637_275000_青森変電所/RConn2 -- L_316581637/LConn2
  L_316581637/LConn3 -- T_316581637_275000_青森変電所/RConn3 -- bus398/LConn1
  T_110682951_275000_宝塚開閉所_(Takarazuka_Kaiheisho)/RConn1 -- L_110682951/LConn1
  T_110682951_275000_宝塚開閉所_(Takarazuka_Kaiheisho)/RConn2 -- L_110682951/LConn2
  L_110682951/LConn3 -- T_110682951_275000_宝塚開閉所_(Takarazuka_Kaiheisho)/RConn3 -- bus399/LConn1
  T_242253497_275000_姫路変電所_(Himeji_Hendensho)/RConn1 -- L_242253497/LConn1
  T_242253497_275000_姫路変電所_(Himeji_Hendensho)/RConn2 -- L_242253497/LConn2
  L_242253497/LConn3 -- T_242253497_275000_姫路変電所_(Himeji_Hendensho)/RConn3 -- bus400/LConn1
  T_185032690_275000_西神戸変電所/RConn1 -- L_185032690/LConn1
  T_185032690_275000_西神戸変電所/RConn2 -- L_185032690/LConn2
  L_185032690/LConn3 -- T_185032690_275000_西神戸変電所/RConn3 -- bus401/LConn1
  T_160374974_275000;77000_北葛城変電所_(Kita_Katsuragi_Hendensho)/RConn1 -- L_160374974/LConn1
  T_160374974_275000;77000_北葛城変電所_(Kita_Katsuragi_Hendensho)/RConn2 -- L_160374974/LConn2
  L_160374974/LConn3 -- T_160374974_275000;77000_北葛城変電所_(Kita_Katsuragi_Hendensho)/RConn3 -- bus402/LConn1
  T_170260161_275000_/RConn1 -- L_170260161/LConn1
  T_170260161_275000_/RConn2 -- L_170260161/LConn2
  L_170260161/LConn3 -- T_170260161_275000_/RConn3 -- bus403/LConn1
  T_170260169_275000_田原/RConn1 -- L_170260169/LConn1
  T_170260169_275000_田原/RConn2 -- L_170260169/LConn2
  L_170260169/LConn3 -- T_170260169_275000_田原/RConn3 -- bus404/LConn1
  T_133644487__/RConn1 -- L_133644487/LConn1
  T_133644487__/RConn2 -- L_133644487/LConn2
  L_133644487/LConn3 -- T_133644487__/RConn3 -- bus405/LConn1
  T_145084773_275000_青梅変電所/RConn1 -- L_145084773/LConn1
  T_145084773_275000_青梅変電所/RConn2 -- L_145084773/LConn2
  L_145084773/LConn3 -- T_145084773_275000_青梅変電所/RConn3 -- bus406/LConn1
  T_159191758_275000_北松本変電所/RConn1 -- L_159191758/LConn1
  T_159191758_275000_北松本変電所/RConn2 -- L_159191758/LConn2
  L_159191758/LConn3 -- T_159191758_275000_北松本変電所/RConn3 -- bus407/LConn1
  T_211258348_275000_東信変電所/RConn1 -- L_211258348/LConn1
  T_211258348_275000_東信変電所/RConn2 -- L_211258348/LConn2
  L_211258348/LConn3 -- T_211258348_275000_東信変電所/RConn3 -- bus408/LConn1
  T_136298957__新座変電所/RConn1 -- L_136298957/LConn1
  T_136298957__新座変電所/RConn2 -- L_136298957/LConn2
  L_136298957/LConn3 -- T_136298957__新座変電所/RConn3 -- bus409/LConn1
  T_199544541_275000_新北信変電所/RConn1 -- L_199544541/LConn1
  T_199544541_275000_新北信変電所/RConn2 -- L_199544541/LConn2
  L_199544541/LConn3 -- T_199544541_275000_新北信変電所/RConn3 -- bus410/LConn1
  T_190734269_275000_/RConn1 -- L_190734269/LConn1
  T_190734269_275000_/RConn2 -- L_190734269/LConn2
  L_190734269/LConn3 -- T_190734269_275000_/RConn3 -- bus411/LConn1
  T_47110637_275000_西東京変電所/RConn1 -- L_47110637/LConn1
  T_47110637_275000_西東京変電所/RConn2 -- L_47110637/LConn2
  L_47110637/LConn3 -- T_47110637_275000_西東京変電所/RConn3 -- bus412/LConn1
  T_291678103_275000_紀の川変電所_(Kinokawa_Hendensho)/RConn1 -- L_291678103/LConn1
  T_291678103_275000_紀の川変電所_(Kinokawa_Hendensho)/RConn2 -- L_291678103/LConn2
  L_291678103/LConn3 -- T_291678103_275000_紀の川変電所_(Kinokawa_Hendensho)/RConn3 -- bus413/LConn1
  T_325868333_275000_/RConn1 -- L_325868333/LConn1
  T_325868333_275000_/RConn2 -- L_325868333/LConn2
  L_325868333/LConn3 -- T_325868333_275000_/RConn3 -- bus414/LConn1
  T_145080115_275000_/RConn1 -- L_145080115/LConn1
  T_145080115_275000_/RConn2 -- L_145080115/LConn2
  L_145080115/LConn3 -- T_145080115_275000_/RConn3 -- bus415/LConn1
  T_308348224_275000_新庄変電所/RConn1 -- L_308348224/LConn1
  T_308348224_275000_新庄変電所/RConn2 -- L_308348224/LConn2
  L_308348224/LConn3 -- T_308348224_275000_新庄変電所/RConn3 -- bus416/LConn1
  T_110682955_275000;154000;77000_伊丹変電所_(Itami_Hendensho)/RConn1 -- L_110682955/LConn1
  T_110682955_275000;154000;77000_伊丹変電所_(Itami_Hendensho)/RConn2 -- L_110682955/LConn2
  L_110682955/LConn3 -- T_110682955_275000;154000;77000_伊丹変電所_(Itami_Hendensho)/RConn3 -- bus417/LConn1
  T_320724312_275000_/RConn1 -- L_320724312/LConn1
  T_320724312_275000_/RConn2 -- L_320724312/LConn2
  L_320724312/LConn3 -- T_320724312_275000_/RConn3 -- bus418/LConn1
  T_316459359_275000_/RConn1 -- L_316459359/LConn1
  T_316459359_275000_/RConn2 -- L_316459359/LConn2
  L_316459359/LConn3 -- T_316459359_275000_/RConn3 -- bus419/LConn1
  T_144077272__/RConn1 -- L_144077272/LConn1
  T_144077272__/RConn2 -- L_144077272/LConn2
  L_144077272/LConn3 -- T_144077272__/RConn3 -- bus420/LConn1
  T_152991099__中東京変電所/RConn1 -- L_152991099/LConn1
  T_152991099__中東京変電所/RConn2 -- L_152991099/LConn2
  L_152991099/LConn3 -- T_152991099__中東京変電所/RConn3 -- bus421/LConn1
  T_190984572_275000_/RConn1 -- L_190984572/LConn1
  T_190984572_275000_/RConn2 -- L_190984572/LConn2
  L_190984572/LConn3 -- T_190984572_275000_/RConn3 -- bus422/LConn1
  T_318302348_275000_東上越変電所/RConn1 -- L_318302348/LConn1
  T_318302348_275000_東上越変電所/RConn2 -- L_318302348/LConn2
  L_318302348/LConn3 -- T_318302348_275000_東上越変電所/RConn3 -- bus423/LConn1
  T_153760214__多摩変電所/RConn1 -- L_153760214/LConn1
  T_153760214__多摩変電所/RConn2 -- L_153760214/LConn2
  L_153760214/LConn3 -- T_153760214__多摩変電所/RConn3 -- bus424/LConn1
  T_315662816__/RConn1 -- L_315662816/LConn1
  T_315662816__/RConn2 -- L_315662816/LConn2
  L_315662816/LConn3 -- T_315662816__/RConn3 -- bus425/LConn1
  T_216778426_500000;220000_/RConn1 -- L_216778426/LConn1
  T_216778426_500000;220000_/RConn2 -- L_216778426/LConn2
  L_216778426/LConn3 -- T_216778426_500000;220000_/RConn3 -- bus426/LConn1
  T_104173570_500000_/RConn1 -- L_104173570/LConn1
  T_104173570_500000_/RConn2 -- L_104173570/LConn2
  L_104173570/LConn3 -- T_104173570_500000_/RConn3 -- bus427/LConn1
  T_168857610__/RConn1 -- L_168857610/LConn1
  T_168857610__/RConn2 -- L_168857610/LConn2
  L_168857610/LConn3 -- T_168857610__/RConn3 -- bus428/LConn1
  T_104530060__新栃木変電所/RConn1 -- L_104530060/LConn1
  T_104530060__新栃木変電所/RConn2 -- L_104530060/LConn2
  L_104530060/LConn3 -- T_104530060__新栃木変電所/RConn3 -- bus429/LConn1
  T_87538349_500000_讃岐変電所/RConn1 -- L_87538349/LConn1
  T_87538349_500000_讃岐変電所/RConn2 -- L_87538349/LConn2
  L_87538349/LConn3 -- T_87538349_500000_讃岐変電所/RConn3 -- bus430/LConn1
  T_171066843_500000_四国電力東予変電所/RConn1 -- L_171066843/LConn1
  T_171066843_500000_四国電力東予変電所/RConn2 -- L_171066843/LConn2
  L_171066843/LConn3 -- T_171066843_500000_四国電力東予変電所/RConn3 -- bus431/LConn1
  T_102958903_500000_/RConn1 -- L_102958903/LConn1
  T_102958903_500000_/RConn2 -- L_102958903/LConn2
  L_102958903/LConn3 -- T_102958903_500000_/RConn3 -- bus432/LConn1
  T_149843487_500000_新秦野変電所_(Shin_Hatano_Hendensho)/RConn1 -- L_149843487/LConn1
  T_149843487_500000_新秦野変電所_(Shin_Hatano_Hendensho)/RConn2 -- L_149843487/LConn2
  L_149843487/LConn3 -- T_149843487_500000_新秦野変電所_(Shin_Hatano_Hendensho)/RConn3 -- bus433/LConn1
  T_145079972_500000_新多摩変電所_(Shin_Tama_Substation)/RConn1 -- L_145079972/LConn1
  T_145079972_500000_新多摩変電所_(Shin_Tama_Substation)/RConn2 -- L_145079972/LConn2
  L_145079972/LConn3 -- T_145079972_500000_新多摩変電所_(Shin_Tama_Substation)/RConn3 -- bus434/LConn1
  T_150035494_500000_/RConn1 -- L_150035494/LConn1
  T_150035494_500000_/RConn2 -- L_150035494/LConn2
  L_150035494/LConn3 -- T_150035494_500000_/RConn3 -- bus435/LConn1
  T_341208725__/RConn1 -- L_341208725/LConn1
  T_341208725__/RConn2 -- L_341208725/LConn2
  L_341208725/LConn3 -- T_341208725__/RConn3 -- bus436/LConn1
  T_66098469_500000_西群馬開閉所/RConn1 -- L_66098469/LConn1
  T_66098469_500000_西群馬開閉所/RConn2 -- L_66098469/LConn2
  L_66098469/LConn3 -- T_66098469_500000_西群馬開閉所/RConn3 -- bus437/LConn1
  T_170589736_500000_東近江/RConn1 -- L_170589736/LConn1
  T_170589736_500000_東近江/RConn2 -- L_170589736/LConn2
  L_170589736/LConn3 -- T_170589736_500000_東近江/RConn3 -- bus438/LConn1
  T_170568495_500000_三重開閉所/RConn1 -- L_170568495/LConn1
  T_170568495_500000_三重開閉所/RConn2 -- L_170568495/LConn2
  L_170568495/LConn3 -- T_170568495_500000_三重開閉所/RConn3 -- bus439/LConn1
  T_116559939_500000_/RConn1 -- L_116559939/LConn1
  T_116559939_500000_/RConn2 -- L_116559939/LConn2
  L_116559939/LConn3 -- T_116559939_500000_/RConn3 -- bus440/LConn1
  T_142662111_500000_中部電力㈱豊根開閉所/RConn1 -- L_142662111/LConn1
  T_142662111_500000_中部電力㈱豊根開閉所/RConn2 -- L_142662111/LConn2
  L_142662111/LConn3 -- T_142662111_500000_中部電力㈱豊根開閉所/RConn3 -- bus441/LConn1
  T_170366035_500000_/RConn1 -- L_170366035/LConn1
  T_170366035_500000_/RConn2 -- L_170366035/LConn2
  L_170366035/LConn3 -- T_170366035_500000_/RConn3 -- bus442/LConn1
  T_170974371_500000_新広島変電所_(Shin_Hiroshima_Hendensho)/RConn1 -- L_170974371/LConn1
  T_170974371_500000_新広島変電所_(Shin_Hiroshima_Hendensho)/RConn2 -- L_170974371/LConn2
  L_170974371/LConn3 -- T_170974371_500000_新広島変電所_(Shin_Hiroshima_Hendensho)/RConn3 -- bus443/LConn1
  T_242253537__開閉所/RConn1 -- L_242253537/LConn1
  T_242253537__開閉所/RConn2 -- L_242253537/LConn2
  L_242253537/LConn3 -- T_242253537__開閉所/RConn3 -- bus444/LConn1
  T_242103481_500000_日野変電所/RConn1 -- L_242103481/LConn1
  T_242103481_500000_日野変電所/RConn2 -- L_242103481/LConn2
  L_242103481/LConn3 -- T_242103481_500000_日野変電所/RConn3 -- bus445/LConn1
  T_241822621_500000_/RConn1 -- L_241822621/LConn1
  T_241822621_500000_/RConn2 -- L_241822621/LConn2
  L_241822621/LConn3 -- T_241822621_500000_/RConn3 -- bus446/LConn1
  T_320438391_500000_/RConn1 -- L_320438391/LConn1
  T_320438391_500000_/RConn2 -- L_320438391/LConn2
  L_320438391/LConn3 -- T_320438391_500000_/RConn3 -- bus447/LConn1
  T_320444665_500000_/RConn1 -- L_320444665/LConn1
  T_320444665_500000_/RConn2 -- L_320444665/LConn2
  L_320444665/LConn3 -- T_320444665_500000_/RConn3 -- bus448/LConn1
  T_315461259_500000_/RConn1 -- L_315461259/LConn1
  T_315461259_500000_/RConn2 -- L_315461259/LConn2
  L_315461259/LConn3 -- T_315461259_500000_/RConn3 -- bus449/LConn1
  T_315608215_500000_/RConn1 -- L_315608215/LConn1
  T_315608215_500000_/RConn2 -- L_315608215/LConn2
  L_315608215/LConn3 -- T_315608215_500000_/RConn3 -- bus450/LConn1
  T_169249243_500000_南福光変電所/RConn1 -- L_169249243/LConn1
  T_169249243_500000_南福光変電所/RConn2 -- L_169249243/LConn2
  L_169249243/LConn3 -- T_169249243_500000_南福光変電所/RConn3 -- bus451/LConn1
  T_169249247_500000_加賀変電所/RConn1 -- L_169249247/LConn1
  T_169249247_500000_加賀変電所/RConn2 -- L_169249247/LConn2
  L_169249247/LConn3 -- T_169249247_500000_加賀変電所/RConn3 -- bus452/LConn1
  T_132913106_500000_新筑波変電所_(Shin_Tsukuba_Hendensho)/RConn1 -- L_132913106/LConn1
  T_132913106_500000_新筑波変電所_(Shin_Tsukuba_Hendensho)/RConn2 -- L_132913106/LConn2
  L_132913106/LConn3 -- T_132913106_500000_新筑波変電所_(Shin_Tsukuba_Hendensho)/RConn3 -- bus453/LConn1
  T_169359724_500000_信貴変電所_(Shingi_Hendensho)/RConn1 -- L_169359724/LConn1
  T_169359724_500000_信貴変電所_(Shingi_Hendensho)/RConn2 -- L_169359724/LConn2
  L_169359724/LConn3 -- T_169359724_500000_信貴変電所_(Shingi_Hendensho)/RConn3 -- bus454/LConn1
  T_317511904_500000_北松江変電所/RConn1 -- L_317511904/LConn1
  T_317511904_500000_北松江変電所/RConn2 -- L_317511904/LConn2
  L_317511904/LConn3 -- T_317511904_500000_北松江変電所/RConn3 -- bus455/LConn1
  T_216956620_500000_/RConn1 -- L_216956620/LConn1
  T_216956620_500000_/RConn2 -- L_216956620/LConn2
  L_216956620/LConn3 -- T_216956620_500000_/RConn3 -- bus456/LConn1
  T_253566674__/RConn1 -- L_253566674/LConn1
  T_253566674__/RConn2 -- L_253566674/LConn2
  L_253566674/LConn3 -- T_253566674__/RConn3 -- bus457/LConn1
  T_104391636_500000_新いわき/RConn1 -- L_104391636/LConn1
  T_104391636_500000_新いわき/RConn2 -- L_104391636/LConn2
  L_104391636/LConn3 -- T_104391636_500000_新いわき/RConn3 -- bus458/LConn1
  T_169963227_500000_新榛名/RConn1 -- L_169963227/LConn1
  T_169963227_500000_新榛名/RConn2 -- L_169963227/LConn2
  L_169963227/LConn3 -- T_169963227_500000_新榛名/RConn3 -- bus459/LConn1
  T_195615141_500000_/RConn1 -- L_195615141/LConn1
  T_195615141_500000_/RConn2 -- L_195615141/LConn2
  L_195615141/LConn3 -- T_195615141_500000_/RConn3 -- bus460/LConn1
  T_169963236__/RConn1 -- L_169963236/LConn1
  T_169963236__/RConn2 -- L_169963236/LConn2
  L_169963236/LConn3 -- T_169963236__/RConn3 -- bus461/LConn1
  T_242103532_500000_/RConn1 -- L_242103532/LConn1
  T_242103532_500000_/RConn2 -- L_242103532/LConn2
  L_242103532/LConn3 -- T_242103532_500000_/RConn3 -- bus462/LConn1
  T_169031922__/RConn1 -- L_169031922/LConn1
  T_169031922__/RConn2 -- L_169031922/LConn2
  L_169031922/LConn3 -- T_169031922__/RConn3 -- bus463/LConn1
  T_169031998__/RConn1 -- L_169031998/LConn1
  T_169031998__/RConn2 -- L_169031998/LConn2
  L_169031998/LConn3 -- T_169031998__/RConn3 -- bus464/LConn1
  T_209429410_500000_南信変電所/RConn1 -- L_209429410/LConn1
  T_209429410_500000_南信変電所/RConn2 -- L_209429410/LConn2
  L_209429410/LConn3 -- T_209429410_500000_南信変電所/RConn3 -- bus465/LConn1
  T_109850439_500000_/RConn1 -- L_109850439/LConn1
  T_109850439_500000_/RConn2 -- L_109850439/LConn2
  L_109850439/LConn3 -- T_109850439_500000_/RConn3 -- bus466/LConn1
  T_217885658_500000;0_由良開閉所/RConn1 -- L_217885658/LConn1
  T_217885658_500000;0_由良開閉所/RConn2 -- L_217885658/LConn2
  L_217885658/LConn3 -- T_217885658_500000;0_由良開閉所/RConn3 -- bus467/LConn1
  T_170605907_500000_北摂変電所/RConn1 -- L_170605907/LConn1
  T_170605907_500000_北摂変電所/RConn2 -- L_170605907/LConn2
  L_170605907/LConn3 -- T_170605907_500000_北摂変電所/RConn3 -- bus468/LConn1
  T_209726348_500000_信濃変電所/RConn1 -- L_209726348/LConn1
  T_209726348_500000_信濃変電所/RConn2 -- L_209726348/LConn2
  L_209726348/LConn3 -- T_209726348_500000_信濃変電所/RConn3 -- bus469/LConn1
  T_315662839_500000_新信濃変電所/RConn1 -- L_315662839/LConn1
  T_315662839_500000_新信濃変電所/RConn2 -- L_315662839/LConn2
  L_315662839/LConn3 -- T_315662839_500000_新信濃変電所/RConn3 -- bus470/LConn1
